simulink model "impedanceControl_current_only"  (Simulink 9.1)
settings: Solver=FixedStepDiscrete  StartTime=0.0  StopTime=Config.SIMULATION_TIME  FixedStep=Config.Ts  RelTol=1e-3  EnableMultiTasking=on
InitFcn:
  | cd(fileparts(which(bdroot)));
  | initImpedanceControl_current_only;
StopFcn:
  | cd(fileparts(which(bdroot)));
  | stopImpedanceControl;
undefined symbols (not defined in the file or in its folder): AMPLS_SETPOINT, Config, CONST_SETPOINT, FREQS_SETPOINT
libraries: WBToolboxLibrary x7
settings Model: SuppressorTable=22 serialization::archive 11 0 6 0 0 0 1 0  Creator=daniele  LastModifiedBy=icub
settings DataIOCC: LimitDataPoints=on
settings DebuggingCC: UnderspecifiedInitializationDetection=Simplified  MergeDetectMultiDrivingBlocksExec=error  SolverPrmCheckMsg=warning  MultiTaskDSMMsg=warning  MultiTaskCondExecSysMsg=none  AllowSymbolicDim=off  StrictBusMsg=ErrorOnBusTreatedAsVector
settings GRTTargetCC: GeneratePreprocessorConditionals=Disable all  CombineOutputUpdateFcns=on  GRTInterface=off

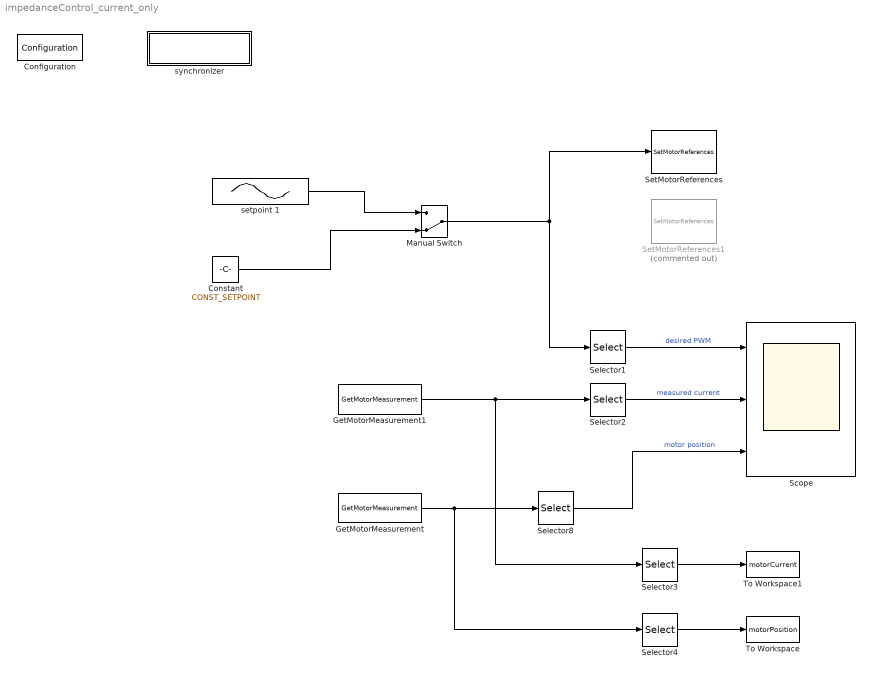
== system impedanceControl_current_only ==
  Configuration : WBToolboxLibrary/Utilities/Configuration  ConfigSource=Workspace  ConfigObject='WBTConfigRobot'
      settings: SourceProductName=WholeBodyToolbox
  Constant : Constant  Value=CONST_SETPOINT
  GetMotorMeasurement : WBToolboxLibrary/States/GetMotorMeasurement  measuredType=Motor Position
      settings: SourceProductName=WholeBodyToolbox
  GetMotorMeasurement1 : WBToolboxLibrary/States/GetMotorMeasurement  measuredType=Motor Current
      settings: SourceProductName=WholeBodyToolbox
  Manual Switch : ManualSwitch  CurrentSetting=0
  Scope : Scope  NumInputPorts=3
  Selector{1..4,8} (5 alike) : Selector  InputPortWidth=ROBOT_DOF  IndexOptions=Index vector (dialog)  Indices=JOINTS_TO_PLOT  OutputSizes=1
  SetMotorReferences : WBToolboxLibrary/Actuators/SetMotorReferences  controlType=PWM
      settings: SourceProductName=WholeBodyToolbox
  SetMotorReferences1 : WBToolboxLibrary/Actuators/SetMotorReferences  Commented=on  controlType=Current
      settings: SourceProductName=WholeBodyToolbox
  To Workspace : ToWorkspace  VariableName=motorPosition  SaveFormat=Timeseries  SampleTime=-1
  To Workspace1 : ToWorkspace  VariableName=motorCurrent  SaveFormat=Timeseries  SampleTime=-1
  setpoint 1 : Sin  Amplitude=AMPLS_SETPOINT  Frequency=FREQS_SETPOINT*2*pi  SampleTime=0
  synchronizer : Subsystem
      mask Display: disp('SYNCHRONIZER')
  wires:
  GetMotorMeasurement/1 -> Selector4/1, Selector8/1
  Selector1/1 -> Scope/1  "desired PWM"
  Selector2/1 -> Scope/2  "measured current"
  Selector8/1 -> Scope/3  "motor position"
  GetMotorMeasurement1/1 -> Selector3/1, Selector2/1
  setpoint 1/1 -> Manual Switch/1
  Constant/1 -> Manual Switch/2
  Manual Switch/1 -> Selector1/1, SetMotorReferences/1
  Selector3/1 -> To Workspace1/1
  Selector4/1 -> To Workspace/1

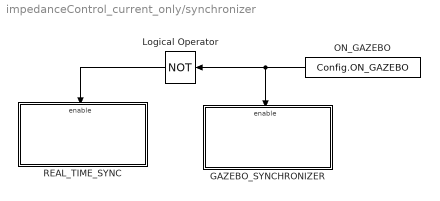
== system impedanceControl_current_only/synchronizer ==
  GAZEBO_SYNCHRONIZER : Subsystem
  Logical Operator : Logic  Operator=NOT  AllPortsSameDT=off  OutDataTypeStr=boolean
  "ON_GAZEBO " : Constant  Value=Config.ON_GAZEBO
  REAL_TIME_SYNC : Subsystem
  wires:
  Logical Operator/1 -> REAL_TIME_SYNC/Enable
  "ON_GAZEBO "/1 -> GAZEBO_SYNCHRONIZER/Enable, Logical Operator/1

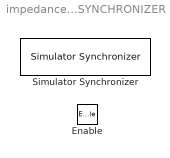
== system impedanceControl_current_only/synchronizer/GAZEBO_SYNCHRONIZER ==
  Enable : EnablePort
  Simulator Synchronizer : WBToolboxLibrary/Utilities/Simulator Synchronizer  period=Config.Ts  serverPortName='/clock/rpc'  clientPortName='/WBT_synchronizer/rpc:o'
      settings: SourceProductName=WholeBodyToolbox

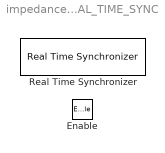
== system impedanceControl_current_only/synchronizer/REAL_TIME_SYNC ==
  Enable : EnablePort
  Real Time Synchronizer : WBToolboxLibrary/Utilities/Real Time Synchronizer  period=Config.Ts
      settings: SourceProductName=WholeBodyToolbox
